simulink model "q_qube2_swingup"  (Simulink 8.3)
settings: Solver=ode1  StartTime=0.0  StopTime=inf  FixedStep=0.002  RelTol=1e-3
values from neighbouring files (symbols this model uses):
  g = 9.81    [qube2_rotpen_param.m]    (also in setup_inverted_pend_ss_model.m; setup_non_inverted_pend_ss_model.m; setup_ss_model.m)
  Jp = Mp*Lp^2/12    (= 3.3282e-05)    [qube2_rotpen_param.m]    (also in setup_inverted_pend_ss_model.m; setup_non_inverted_pend_ss_model.m; setup_ss_model.m)
  kt = 0.042    [qube2_rotpen_param.m]    (also in setup_inverted_pend_ss_model.m; setup_non_inverted_pend_ss_model.m; setup_ss_model.m)
  Lp = 0.129    [qube2_rotpen_param.m]    (also in setup_inverted_pend_ss_model.m; setup_non_inverted_pend_ss_model.m; setup_ss_model.m)
  Lr = 0.085    [qube2_rotpen_param.m]    (also in setup_inverted_pend_ss_model.m; setup_non_inverted_pend_ss_model.m; setup_ss_model.m)
  Mp = 0.024    [qube2_rotpen_param.m]    (also in setup_inverted_pend_ss_model.m; setup_non_inverted_pend_ss_model.m; setup_ss_model.m)
  Mr = 0.095    [qube2_rotpen_param.m]    (also in setup_inverted_pend_ss_model.m; setup_non_inverted_pend_ss_model.m; setup_ss_model.m)
  Rm = 8.4    [qube2_rotpen_param.m]    (also in setup_inverted_pend_ss_model.m; setup_non_inverted_pend_ss_model.m; setup_ss_model.m)
undefined symbols (not defined in the file or in its folder): HIL, qc_get_step_size
libraries: simulink x4, quarc_library x3, simulink_extras x2
settings Model: Creator=MLevis  LastModifiedBy=mbohra  SimulationMode=external  ExtModeTrigDuration=5000  BufferReuse=off
settings SolverCC: PositivePriorityOrder=on
settings OptimizationCC: BooleanDataType=off  OptimizeBlockIOStorage=off  BufferReuse=off  GlobalBufferReuse=off  ExpressionFolding=off  ExpressionDepthLimit=2147483647  LocalBlockOutputs=off  InitFltsAndDblsToZero=on
settings DebuggingCC: SaveWithParameterizedLinksMsg=none  SignalResolutionControl=TryResolveAllWithWarning  SolverPrmCheckMsg=none  MultiTaskDSMMsg=warning  MultiTaskCondExecSysMsg=none  FcnCallInpInsideContextMsg=UseLocalSettings
settings HardwareCC: TargetHWDeviceType=32-bit Generic
settings SFSimCC: SimParseCustomCode=off
settings RTWCC: SystemTargetFile=quarc_win64.tlc  TemplateMakefile=quarc_default_tmf  Description=QUARC Win64 Target  ProcessScript=quarc_win64_make_rtw_hook  IncludeERTFirstTime=on
settings STFCustomTargetCC: TargetPreCompLibLocation=C:\PROGRA~3\QUARC\lib\2014a\win64\release  ConcurrentExecutionCompliant=on  GeneratePreprocessorConditionals=Disable all  CPPClassGenCompliant=on  SystemTargetFile=quarc_win64.tlc
settings GRTTargetCC: TargetPreCompLibLocation=C:\PROGRA~3\QUARC\lib\2014a\win64\release  ParMdlRefBuildCompliant=off  CompOptLevelCompliant=off  MatFileLogging=off  ExtMode=on  ExtModeMexFile=quarc_comm

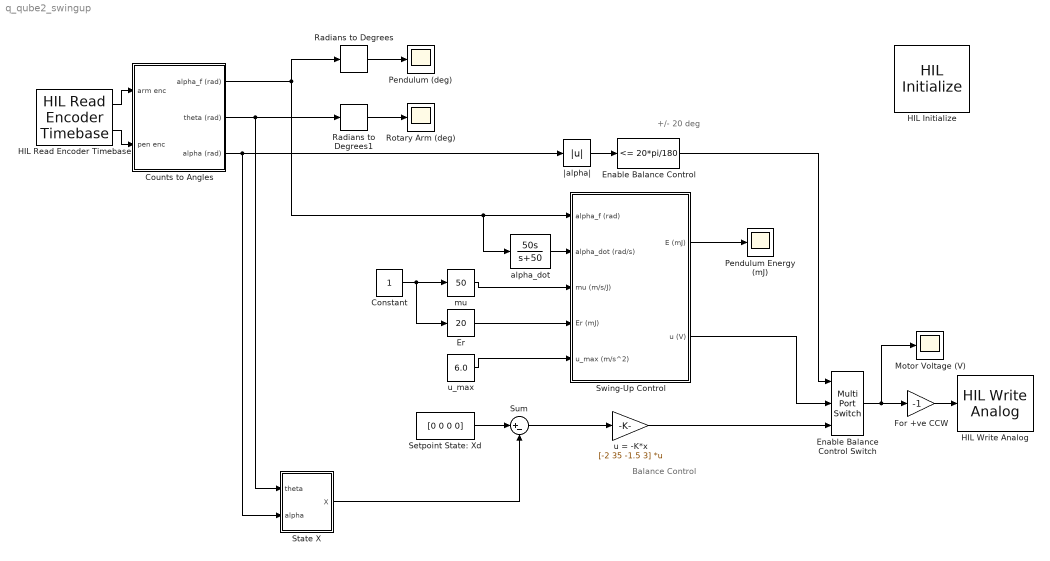
== system q_qube2_swingup ==
  note: +/- 20 deg
  note: Balance Control
  Constant : Constant
  Counts to Angles : Subsystem
  Enable Balance Control : simulink/Logic and Bit Operations/Compare To Constant  relop=<=  const=20*pi/180  OutDataTypeStr=uint8  ZeroCross=off
  Enable Balance Control Switch : MultiPortSwitch  DataPortOrder=Zero-based contiguous  Inputs=2  zeroidx=on
  Er : simulink/Math Operations/Slider Gain  low=0  gain=20  high=50
  For +ve CCW : Gain  Gain=-1
  HIL Initialize : quarc_library/Data Acquisition/Generic/Configuration/HIL Initialize  object_name=HIL-1  board_type=qube_servo2_usb  board_number=0  board_options=""  exclusive=off  active=off  hardware_clocks=[0]  clock_modes=[]  initial_clock_frequencies=[]  set_clock_params_at_start=off  set_clock_params_at_switch_in=off  set_clock_frequencies_at_start=off  set_clock_frequencies_at_switch_in=off  analog_input_channels=[0]  analog_input_maximums=3  analog_input_minimums=-3  set_analog_input_params_at_start=off  set_analog_input_params_at_switch_in=off  analog_output_channels=[0]  analog_output_maximums=15  analog_output_minimums=-15  initial_analog_outputs=[0]  final_analog_outputs=[0]  watchdog_analog_outputs=0  set_analog_output_params_at_start=off  set_analog_output_params_at_switch_in=off  set_analog_outputs_at_start=on  set_analog_outputs_at_switch_in=off  set_analog_outputs_at_terminate=on  set_analog_outputs_at_switch_out=off  set_analog_outputs_on_watchdog=on  digital_input_channels=[]  digital_output_channels=[0]  digital_output_configuration=[]  initial_digital_outputs=[1]  final_digital_outputs=[0]  watchdog_digital_outputs=[0]  set_digital_output_params_at_start=off  set_digital_output_params_at_switch_in=off  set_digital_outputs_at_start=on  set_digital_outputs_at_switch_in=off  set_digital_outputs_at_terminate=on  set_digital_outputs_at_switch_out=off  set_digital_outputs_on_watchdog=on  encoder_channels=[0:1]  quadrature=[4]  encoder_filter_frequency=[]  initial_encoder_counts=[0]  set_encoder_params_at_start=off  set_encoder_params_at_switch_in=off  set_encoder_counts_at_start=on  set_encoder_counts_at_switch_in=off  pwm_channels=[]  pwm_modes=[]  pwm_frequency=[]  pwm_configuration=[]  pwm_alignment=[]  pwm_polarity=[]  pwm_leading_deadband=[]  pwm_trailing_deadband=[]  initial_pwm_outputs=[]  final_pwm_outputs=[]  watchdog_pwm_outputs=[]  set_pwm_params_at_start=off  set_pwm_params_at_switch_in=off  set_pwm_outputs_at_start=off  set_pwm_outputs_at_switch_in=off  set_pwm_outputs_at_terminate=off  set_pwm_outputs_at_switch_out=off  set_pwm_outputs_on_watchdog=off  other_output_channels=[11000:11002]  initial_other_outputs=[0 1 0]  final_other_outputs=[1 0 0]  watchdog_other_outputs=[0 0 1]  set_other_outputs_at_start=on  set_other_outputs_at_switch_in=off  set_other_outputs_at_terminate=on  set_other_outputs_at_switch_out=off  set_other_outputs_on_watchdog=on
  HIL Read Encoder Timebase : quarc_library/Data Acquisition/Generic/Timebases/HIL Read Encoder Timebase  object_name=HIL-1  clock=0  channels=[0:1]  samples_in_buffer=max(ceil(1/qc_get_step_size), 1)  active=on  vector_output=off  data_type_mode=Inherit via back propagation  data_type=double
  HIL Write Analog : quarc_library/Data Acquisition/Generic/Immediate I//O/HIL Write Analog  object_name=HIL-1  channels=0  sample_time=-1  active=off  vector_input=off
  Motor Voltage (V) : Scope
      settings: TimeRange=10  YMin=-12.5  YMax=12.5
  Pendulum (deg) : Scope
      settings: TimeRange=10  YMin=-200  YMax=200  SaveName=ScopeData2
  Pendulum Energy (mJ) : Scope
      settings: TimeRange=10  YMin=0  YMax=50  SaveName=ScopeData3
  Radians to Degrees : simulink_extras/Transformations/Radians to Degrees
  Radians to Degrees1 : simulink_extras/Transformations/Radians to Degrees
  Rotary Arm (deg) : Scope
      settings: TimeRange=10  YMin=-90  YMax=90
  Setpoint State: Xd : Constant  Value=[0 0 0 0]
  State X : Subsystem
  Sum : Sum  Inputs=|+-
  Swing-Up Control : Subsystem
  alpha_dot : TransferFcn  Numerator=[50 0]  Denominator=[1 50]
  mu : simulink/Math Operations/Slider Gain  low=0  gain=50  high=100
  u = -K*x : Gain  Gain=[-2 35 -1.5 3]  Multiplication=Matrix(K*u)
  u_max : Constant  Value=6.0
  |alpha| : Abs
  wires:
  |alpha|/1 -> Enable Balance Control/1
  Swing-Up Control/2(u (V)) -> Enable Balance Control Switch/2
  Constant/1 -> mu/1, Er/1
  mu/1 -> Swing-Up Control/3(mu (m/s/J))
  u_max/1 -> Swing-Up Control/5(u_max (m/s^2))
  For +ve CCW/1 -> HIL Write Analog/1
  HIL Read Encoder Timebase/1 -> Counts to Angles/1(arm enc)
  HIL Read Encoder Timebase/2 -> Counts to Angles/2(pen enc)
  Counts to Angles/2(theta (rad)) -> Radians to Degrees1/1, State X/1(theta)
  Counts to Angles/1(alpha_f (rad)) -> Radians to Degrees/1, Swing-Up Control/1(alpha_f (rad)), alpha_dot/1
  Counts to Angles/3(alpha (rad)) -> |alpha|/1, State X/2(alpha)
  Enable Balance Control/1 -> Enable Balance Control Switch/1
  Sum/1 -> u = -K*x/1
  u = -K*x/1 -> Enable Balance Control Switch/3
  State X/1(X) -> Sum/2
  Setpoint State: Xd/1 -> Sum/1
  Radians to Degrees/1 -> Pendulum (deg)/1
  Radians to Degrees1/1 -> Rotary Arm (deg)/1
  Er/1 -> Swing-Up Control/4(Er (mJ))
  alpha_dot/1 -> Swing-Up Control/2(alpha_dot (rad/s))
  Swing-Up Control/1(E (mJ)) -> Pendulum Energy (mJ)/1
  Enable Balance Control Switch/1 -> For +ve CCW/1, Motor Voltage (V)/1

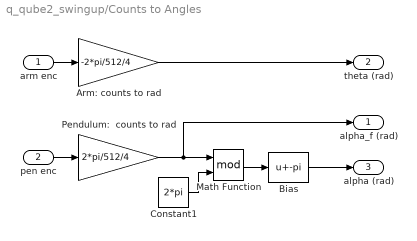
== system q_qube2_swingup/Counts to Angles ==
  arm enc : Inport
  pen enc : Inport  Port=2
  Arm: counts to rad : Gain  Gain=-2*pi/512/4
  Bias : Bias  Bias=-pi
  Constant1 : Constant  Value=2*pi
  Math Function : Math  Operator=mod  SaturateOnIntegerOverflow=on
  Pendulum:  counts to rad : Gain  Gain=2*pi/512/4
  alpha_f (rad) : Outport
  theta (rad) : Outport  Port=2
  alpha (rad) : Outport  Port=3
  wires:
  pen enc/1 -> Pendulum:  counts to rad/1
  arm enc/1 -> Arm: counts to rad/1
  Math Function/1 -> Bias/1
  Constant1/1 -> Math Function/2
  Pendulum:  counts to rad/1 -> Math Function/1, alpha_f (rad)/1
  Arm: counts to rad/1 -> theta (rad)/1
  Bias/1 -> alpha (rad)/1

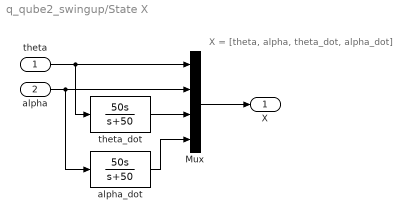
== system q_qube2_swingup/State X ==
  note: X = [theta, alpha, theta_dot, alpha_dot]
  theta : Inport
  alpha : Inport  Port=2
  Mux : Mux
  alpha_dot : TransferFcn  Numerator=[50 0]  Denominator=[1 50]
  theta_dot : TransferFcn  Numerator=[50 0]  Denominator=[1 50]
  X : Outport
  wires:
  theta_dot/1 -> Mux/3
  alpha_dot/1 -> Mux/4
  alpha/1 -> Mux/2, alpha_dot/1
  Mux/1 -> X/1
  theta/1 -> Mux/1, theta_dot/1

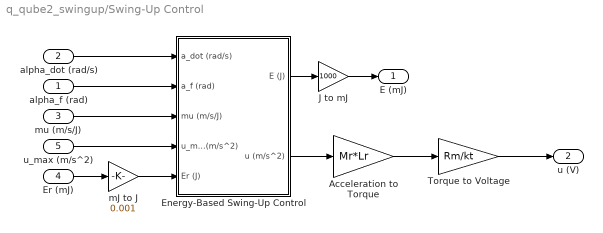
== system q_qube2_swingup/Swing-Up Control ==
  alpha_f (rad) : Inport
  alpha_dot (rad/s) : Inport  Port=2
  mu (m/s/J) : Inport  Port=3
  Er (mJ) : Inport  Port=4
  u_max (m/s^2) : Inport  Port=5
  Acceleration to Torque : Gain  Gain=Mr*Lr
  Energy-Based Swing-Up Control : Subsystem
  J to mJ : Gain  Gain=1000
  Torque to Voltage : Gain  Gain=Rm/kt
  mJ to J : Gain  Gain=0.001
  E (mJ) : Outport
  u (V) : Outport  Port=2
  wires:
  Energy-Based Swing-Up Control/2(u (m/s^2)) -> Acceleration to Torque/1
  Energy-Based Swing-Up Control/1(E (J)) -> J to mJ/1
  alpha_f (rad)/1 -> Energy-Based Swing-Up Control/2(a_f (rad))
  mu (m/s/J)/1 -> Energy-Based Swing-Up Control/3(mu (m/s/J))
  u_max (m/s^2)/1 -> Energy-Based Swing-Up Control/4(u_max (m/s^2))
  Torque to Voltage/1 -> u (V)/1
  Acceleration to Torque/1 -> Torque to Voltage/1
  alpha_dot (rad/s)/1 -> Energy-Based Swing-Up Control/1(a_dot (rad/s))
  Er (mJ)/1 -> mJ to J/1
  mJ to J/1 -> Energy-Based Swing-Up Control/5(Er (J))
  J to mJ/1 -> E (mJ)/1

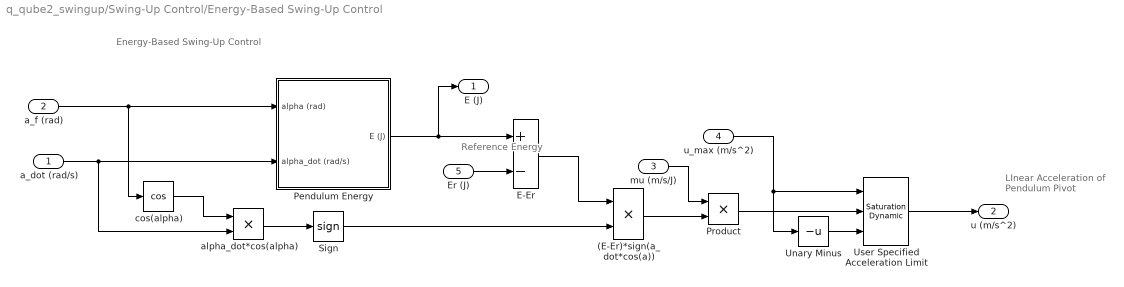
== system q_qube2_swingup/Swing-Up Control/Energy-Based Swing-Up Control ==
  note: Energy-Based Swing-Up Control
  note: LInear Acceleration of
      | Pendulum Pivot
  note: Reference Energy
  a_dot (rad/s) : Inport
  a_f (rad) : Inport  Port=2
  mu (m/s/J) : Inport  Port=3
  u_max (m/s^2) : Inport  Port=4
  Er (J) : Inport  Port=5
  (E-Er)*sign(a_dot*cos(a)) : Product  RndMeth=Zero
  E-Er : Sum  Inputs=+-
  Pendulum Energy : Subsystem
  Product : Product  RndMeth=Zero
  Sign : Signum
  Unary Minus : UnaryMinus
  User Specified Acceleration Limit : simulink/Discontinuities/Saturation Dynamic  OutMin=[]  OutMax=[]  OutDataTypeStr=Inherit: Same as second input  OutDataType=fixdt(1, 16)  OutScaling=2^-10  DoSatur=off
  alpha_dot*cos(alpha) : Product  RndMeth=Zero
  cos(alpha) : Trigonometry  Operator=cos
  E (J) : Outport
  u (m/s^2) : Outport  Port=2
  wires:
  alpha_dot*cos(alpha)/1 -> Sign/1
  Sign/1 -> (E-Er)*sign(a_dot*cos(a))/2
  cos(alpha)/1 -> alpha_dot*cos(alpha)/1
  a_f (rad)/1 -> cos(alpha)/1, Pendulum Energy/1(alpha (rad))
  E-Er/1 -> (E-Er)*sign(a_dot*cos(a))/1
  Pendulum Energy/1(E (J)) -> E (J)/1, E-Er/1
  a_dot (rad/s)/1 -> alpha_dot*cos(alpha)/2, Pendulum Energy/2(alpha_dot (rad/s))
  (E-Er)*sign(a_dot*cos(a))/1 -> Product/2
  Er (J)/1 -> E-Er/2
  mu (m/s/J)/1 -> Product/1
  Product/1 -> User Specified Acceleration Limit/2
  u_max (m/s^2)/1 -> User Specified Acceleration Limit/1, Unary Minus/1
  Unary Minus/1 -> User Specified Acceleration Limit/3
  User Specified Acceleration Limit/1 -> u (m/s^2)/1

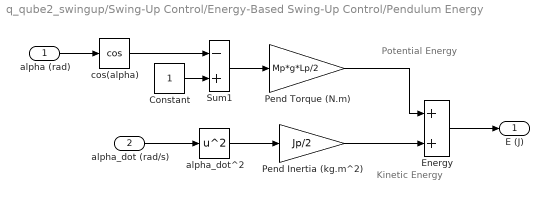
== system q_qube2_swingup/Swing-Up Control/Energy-Based Swing-Up Control/Pendulum Energy ==
  note: Kinetic Energy
  note: Potential Energy
  alpha (rad) : Inport
  alpha_dot (rad/s) : Inport  Port=2
  Constant : Constant
  Energy : Sum  SaturateOnIntegerOverflow=on
  Pend Inertia (kg.m^2) : Gain  Gain=Jp/2
  Pend Torque (N.m) : Gain  Gain=Mp*g*Lp/2
  Sum1 : Sum  Inputs=-+  SaturateOnIntegerOverflow=on
  alpha_dot^2 : Math  Operator=square  SaturateOnIntegerOverflow=on
  cos(alpha) : Trigonometry  Operator=cos
  E (J) : Outport
  wires:
  Constant/1 -> Sum1/2
  Pend Inertia (kg.m^2)/1 -> Energy/2
  Sum1/1 -> Pend Torque (N.m)/1
  alpha_dot^2/1 -> Pend Inertia (kg.m^2)/1
  Pend Torque (N.m)/1 -> Energy/1
  alpha (rad)/1 -> cos(alpha)/1
  alpha_dot (rad/s)/1 -> alpha_dot^2/1
  Energy/1 -> E (J)/1
  cos(alpha)/1 -> Sum1/1
